simulink model "robot"  (R2023b)
settings: Solver=FixedStepAuto  StartTime=0.0  StopTime=20  FixedStep=0.1  RelTol=1e-3
settings Model: Creator=fuxa9  LastModifiedBy=fuxa9

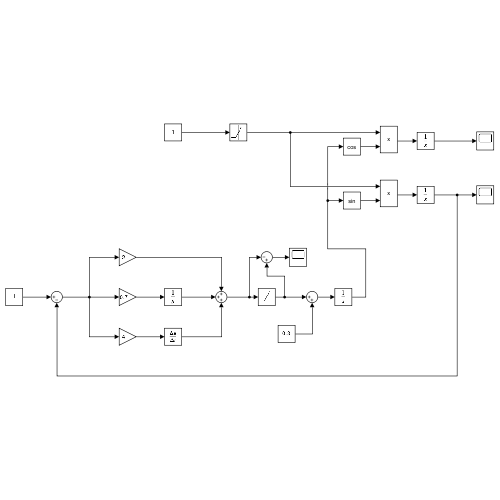
[thumbnail: Simulink's stored preview of the top-level diagram]
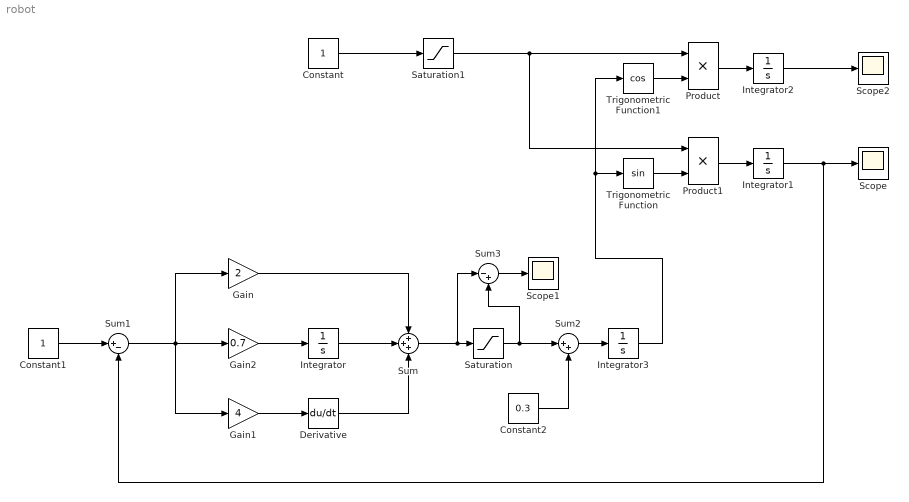
== system robot ==
  Constant : Constant
  Constant1 : Constant
  Constant2 : Constant  Value=0.3
  Derivative : Derivative
  Gain : Gain  Gain=2
  Gain1 : Gain  Gain=4
  Gain2 : Gain  Gain=0.7
  Integrator{,1..3} (4 alike) : Integrator
  Product : Product
  Product1 : Product
  Saturation : Saturate  UpperLimit=2  LowerLimit=-2
  Saturation1 : Saturate  UpperLimit=1  LowerLimit=-1
  Scope : Scope
  Scope1 : Scope
  Scope2 : Scope
  Sum : Sum  Inputs=+++
  Sum1 : Sum  Inputs=|+-
  Sum2 : Sum  Inputs=|++
  Sum3 : Sum  Inputs=|-+
  Trigonometric Function : Trigonometry
  Trigonometric Function1 : Trigonometry  Operator=cos
  wires:
  Gain2/1 -> Integrator/1
  Integrator/1 -> Sum/2
  Gain/1 -> Sum/1
  Gain1/1 -> Derivative/1
  Derivative/1 -> Sum/3
  Sum1/1 -> Gain1/1, Gain/1, Gain2/1
  Product/1 -> Integrator2/1
  Sum2/1 -> Integrator3/1
  Integrator3/1 -> Trigonometric Function1/1, Trigonometric Function/1
  Trigonometric Function/1 -> Product1/2
  Trigonometric Function1/1 -> Product/2
  Sum/1 -> Sum3/1, Saturation/1
  Saturation/1 -> Sum3/2, Sum2/1
  Saturation1/1 -> Product1/1, Product/1
  Constant/1 -> Saturation1/1
  Integrator1/1 -> Sum1/2, Scope/1
  Constant1/1 -> Sum1/1
  Constant2/1 -> Sum2/2
  Sum3/1 -> Scope1/1
  Product1/1 -> Integrator1/1
  Integrator2/1 -> Scope2/1
